simulink model "boost_ms"  (R2020b)
settings: Solver=VariableStepAuto  StartTime=0.0  StopTime=10.0  RelTol=1e-3
libraries: powerlib x10, powerlib_meascontrol x3, re_lib x1
settings Model: Creator=mcapuano  LastModifiedBy=mcapuano

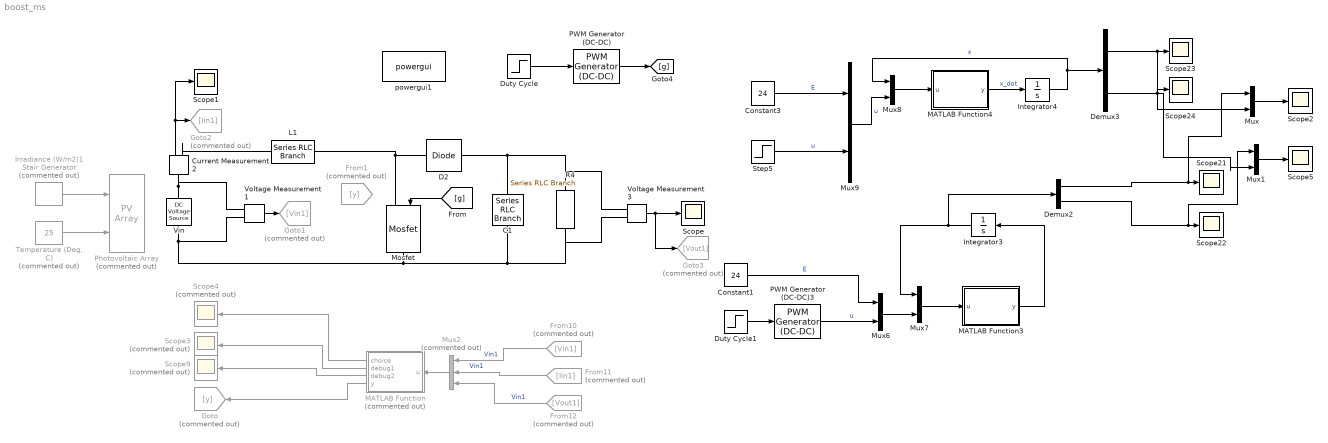
== system boost_ms ==
  C1 : powerlib/Elements/Series RLC Branch  LConnTagsString=__new0  RConnTagsString=__new0  BranchType=C  Resistance=1e-4  Inductance=200e-6  SetiL0=off  InitialCurrent=0  Capacitance=200e-6  Setx0=on  InitialVoltage=0  Measurements=None
  Constant1 : Constant  Value=24
  Constant3 : Constant  Value=24
  Current Measurement2 : powerlib/Measurements/Current Measurement  PhasorSimulation=off  OutputType=Complex  PSBequivalent=0
  D2 : powerlib/Power Electronics/Diode  Ron=1e-3  Lon=0  Vf=0  IC=0  UseSnubber=off  Rs=inf  Cs=inf  Measurements=off
  Demux2 : Demux  Outputs=2
  Demux3 : Demux  Outputs=2
  Duty Cycle : Step  Time=.5  Before=.5  After=.5  SampleTime=0
  Duty Cycle1 : Step  Time=.1  Before=.5  After=.5  SampleTime=0
  From1 : From  Commented=on  GotoTag=y
  From10 : From  Commented=on  GotoTag=Vin1
  From11 : From  Commented=on  GotoTag=Iin1
  From12 : From  Commented=on  GotoTag=Vout1
  Goto : Goto  Commented=on  GotoTag=y
  Goto1 : Goto  Commented=on  GotoTag=Vin1
  Goto2 : Goto  Commented=on  GotoTag=Iin1
  Goto3 : Goto  Commented=on  GotoTag=Vout1
  Integrator3 : Integrator  InitialCondition=[0 0]
  Integrator4 : Integrator  InitialCondition=[0 0]
  Irradiance (W/m2)1 : powerlib_meascontrol/Pulse & Signal Generators/Stair Generator  Commented=on  t=[0, 0.5, 1, 1.5, 2]  e=[0.5, 0.7, 0.8, 0.6, 0.2]*1000  Ts=15e-6
  L1 : powerlib/Elements/Series RLC Branch  LConnTagsString=__new0  RConnTagsString=__new0  BranchType=L  Resistance=1e-4  Inductance=250e-6  SetiL0=on  InitialCurrent=0  Capacitance=30e-6  Setx0=off  InitialVoltage=150  Measurements=None
  MATLAB Function : MATLAB Function  Commented=on  TreatAsAtomicUnit=on  SystemSampleTime=15e-6
  MATLAB Function3 : MATLAB Function  TreatAsAtomicUnit=on
  MATLAB Function4 : MATLAB Function  TreatAsAtomicUnit=on
  Mosfet : powerlib/Power Electronics/Mosfet  Ron=1e-3  Lon=0  Rd=1e-3  Vfd=0  IC=0  Rs=1e6  Cs=inf  Measurements=off
  Mux{,1,6..9} (6 alike) : Mux  Inputs=2
  Mux2 : Mux  Commented=on  Inputs=3
  PWM Generator (DC-DC) : powerlib_meascontrol/Pulse & Signal Generators/PWM Generator (DC-DC)  Fsw=66.67e3  Ts=0
  PWM Generator (DC-DC)3 : powerlib_meascontrol/Pulse & Signal Generators/PWM Generator (DC-DC)  Fsw=66.67e3  Ts=0
  Photovoltaic Array : re_lib/Solar/PV Array  Commented=on  Npar=1  Nser=1  PlotType=one module @ 25 deg.C & specified irradiances  S_vec=[800]  Temp_C_vec=[ 50 ]  ModuleName=Kyocera Solar KC200GT  PlotWhenSelected=off  Pm=200.143  Ncell=54  Voc=32.9  Isc=8.21  Vm=26.3  Im=7.61  beta_Voc_pc=-0.355  alpha_Isc_pc=0.06  beta_Voc=-0.11679  alpha_Isc=0.004926  IL=8.2288  I0=2.3234e-10  nI=0.97734  Rsh=150.6844  Rs=0.34484  RobustModel=off  RobustCellTemperature=313.3991  BAL=on  Tc=1e-6  Tfilter=5e-5
      settings: AttributesFormatString=|
      | %<ModuleName>
      | %<Nser>-module string
      | %<Npar> parallel strings
  R4 : powerlib/Elements/Series RLC Branch  LConnTagsString=__new0  RConnTagsString=__new0  BranchType=R  Resistance=3  Inductance=200e-6  SetiL0=off  InitialCurrent=0  Capacitance=400e-6  Setx0=off  InitialVoltage=0  Measurements=None
  Scope{,1..2,5,21..24} (8 alike) : Scope
  Scope3 : Scope  Commented=on
  Scope4 : Scope  Commented=on
  Scope9 : Scope  Commented=on
  Step5 : Step  Time=.1  Before=.5  After=.5  SampleTime=0
  Temperature (Deg. C) : Constant  Commented=on  Value=25
  Vin : powerlib/Electrical Sources/DC Voltage Source  Amplitude=24  Measurements=None
  Voltage Measurement1 : powerlib/Measurements/Voltage Measurement  PhasorSimulation=off  OutputType=Complex  PSBequivalent=0
  Voltage Measurement3 : powerlib/Measurements/Voltage Measurement  PhasorSimulation=off  OutputType=Complex  PSBequivalent=0
  powergui1 : powerlib/powergui  Priority=1  SimulationMode=Continuous  SampleTime=50e-6  frequency=60  Iterations=50  frequencyindice=0  Pbase=100e6  ErrMax=1e-4  UnitsV=kV  UnitsW=MW  buscounter=0  FunctionMessages=off  echomessages=off  EnableUseOfTLC=off  CurrentSourceSwitches=off  DisableSnubberDevices=off  DisableRonSwitches=off  DisableVfSwitches=off  DisplayEquations=off  AutomaticDiscreteSolvers=off  SolverType=Tustin/Backward Euler (TBE)  Interpol=off  ExternalGateDelay=off  methode=off  Ts=100  x0status=blocks  SPID=on  SwTol=0  HookPort=off  NonlinearTolerance=1e-4  nMaxIteration=100  ContinueOnMaxIteration=off  RestoreLinks=warning  ResistiveCurrentMeasurement=off  Frange=[0:2:500]  Ylog=off  Xlog=on  ShowGrid=off  save=off  variable=ZData  structure=0  ZoomFFT=off  StartTime=0.0  cycles=1  DisplayStyle=1  fundamental=60  FreqAxis=off  MaxFrequency=1000  frequencyindicesteady=1  RmsSteady=1  display=off
  wires:
  PWM Generator (DC-DC)/1 -> [g]
  Duty Cycle/1 -> PWM Generator (DC-DC)/1
  [g] -> Mosfet/1
  Voltage Measurement3/1 -> Goto3/1, Scope/1
  Temperature (Deg. C)/1 -> Photovoltaic Array/2
  Irradiance (W/m2)1/1 -> Photovoltaic Array/1
  MATLAB Function/3(debug2) -> Scope9/1
  From11/1 -> Mux2/2  "Vin1"
  MATLAB Function/2(debug1) -> Scope3/1
  MATLAB Function/1(choice) -> Scope4/1
  From10/1 -> Mux2/1  "Vin1"
  Mux2/1 -> MATLAB Function/1(u)
  From12/1 -> Mux2/3  "Vin1"
  MATLAB Function/4(y) -> Goto/1
  Voltage Measurement1/1 -> Goto1/1
  Current Measurement2/1 -> Scope1/1, Goto2/1
  Mux9/1 -> Mux8/2  "u"
  Constant3/1 -> Mux9/1  "E"
  Demux2/2 -> Mux1/1, Scope22/1
  PWM Generator (DC-DC)3/1 -> Mux6/2  "u"
  Mux8/1 -> MATLAB Function4/1(u)
  Integrator3/1 -> Demux2/1, Mux7/1
  Demux3/1 -> Mux/2, Scope23/1
  Mux7/1 -> MATLAB Function3/1(u)
  Integrator4/1 -> Mux8/1, Demux3/1  "x"
  Demux3/2 -> Mux1/2, Scope24/1
  Mux6/1 -> Mux7/2
  Demux2/1 -> Mux/1, Scope21/1
  Duty Cycle1/1 -> PWM Generator (DC-DC)3/1
  MATLAB Function4/1(y) -> Integrator4/1  "x_dot"
  MATLAB Function3/1(y) -> Integrator3/1
  Constant1/1 -> Mux6/1  "E"
  Step5/1 -> Mux9/2  "u"
  Mux/1 -> Scope2/1
  Mux1/1 -> Scope5/1
  connections:
  Vin/RConn1 -- Voltage Measurement1/LConn1 -- Current Measurement2/LConn1
  Vin/LConn1 -- Voltage Measurement1/LConn2 -- Voltage Measurement3/LConn2 -- R4/RConn1 -- C1/RConn1 -- Mosfet/RConn1
  L1/RConn1 -- Mosfet/LConn1 -- D2/LConn1
  D2/RConn1 -- Voltage Measurement3/LConn1 -- R4/LConn1 -- C1/LConn1
  Current Measurement2/RConn1 -- L1/LConn1

== matlab function boost_ms/MATLAB Function ==
  settings: updateMethod=DISCRETE
  data: choice output; debug1 output; debug2 output; u input; y output
function [choice, debug1, debug2, y]= fcn(u)
Vpv=u(1);
Ipv=u(2);
Vout=u(3);

%This module contains the MPC-MPPT Control Algorithm

%The MPC module follows the flow chart of Fig. 8 in Referenced Research Paper

%This MATLAB fn block's settings have been changed to have a sampling rate
%of 15uS instead of being continous sample mode


%prevent crazy simulation transients from breaking the algorithm:
if (Ipv > 10)
    Ipv = 1;
end

persistent Vpv_t_1; %previous Vpv Sample
if isempty(Vpv_t_1)
    Vpv_t_1 = 0;
end
persistent Ipv_t_1; %previous Ipv Sample
if isempty(Ipv_t_1)
    Ipv_t_1 = 0;
end
persistent Dpv_t_1; % Iref (output) value from what is now 2 timesteps ago
if isempty(Dpv_t_1)
    Dpv_t_1 = 0;
end
persistent Dpv;  %Previous / Most recent Iref (output) Calc
if isempty(Dpv)
    Dpv = 0;
end

Ts = 15e-6; %sample rate
L = 3e-3; %inductance


delta_V = Vpv - Vpv_t_1;
delta_I = Ipv - Ipv_t_1;
delta_D = Dpv - Dpv_t_1;


%fixed vs adaptive
scale_factor_C = 10; %increase for larger output increments/swings
 Z =.01; %fixed 
%Z = scale_factor_C * abs(delta_I * delta_D); %adaptive

% custom adaptive to fix issues with no change causing 0 step size
 adapZ = scale_factor_C * abs(delta_I * delta_D);
% if(adapZ > .1)
%     Z = .1;
% elseif(adapZ > .001)
%     Z = adapZ;
% else
%     Z = .001;
% end

Ipred_1 = Ipv + 2*(Ts/L) * Vpv; %MPC prediction for switch = 1
Ipred_0 = Ipv + (Ts/(2*L)* (Vpv - Vout)); %MPC prediction for switch = 0 

if delta_V == 0 %Inc. Cond. Algo to determin Iref
    if delta_I == 0 
        Iref = Dpv; choice = 0;
    else
        if delta_I > 0
            Iref = Dpv - Z; choice = 1;
        else
            Iref = Dpv + Z; choice = 2;
        end
    end
else
    if (Ipv + (delta_I/delta_V) * Vpv) == 0
        Iref = Dpv; choice = 3;
    else
        if (Ipv + (delta_I/delta_V) * Vpv) > 0
            Iref = Dpv - Z; choice = 4;
        else
            Iref = Dpv + Z; choice = 5;
        end
    end
end

G1 = abs(Iref - Ipred_1); %Optimize MPC by applying Iref
G0 = abs(Iref - Ipred_0);
if G1 < G0
    y = 1;
else
    y = 0;
end

if (Iref < 0)
    Iref = .001;
end
%test = Ipv + (delta_I/delta_V) * Vpv;
test =  delta_V;
%update static variables here:
Vpv_t_1 = Vpv; %previous Vpv Sample
Ipv_t_1 = Ipv; %previous Ipv Sample
Dpv_t_1 = Dpv; % Iref (output) value from what is now 2 timesteps ago
Dpv = Iref;  %Previous / Most recent Iref (output) Calc

%debug purposes:
debug1 = Vout;
debug2 = delta_I/delta_V;

== matlab function boost_ms/MATLAB Function3 ==
  data: u input; y output
function y = fcn(u)
X=u(1:2);
E=u(3);
u=u(4);
% parameters:
C=200e-6;
L=250e-6;
R=3;

% Compact form
A=[ 0    -1/L ;
   1/C  -1/(C*R)];

B=[0   1/L;
   -1/C  0];

b=[0; 0];

d=[E/L; 0];

y = A*X+(B*X+ b)*u+d;

== matlab function boost_ms/MATLAB Function4 ==
  data: u input; y output
function y = fcn(u)

X=u(1:2);
E=u(3);
u=u(4);
% parameters:
C=200e-6;
L=250e-6;
R=3;

%%%begin PWM detector
% persistent D; 
% if isempty(D)
%     D = 0;
% end
% 
% persistent T_on; 
% if isempty(T_on)
%     T_on = 0;
% end
% 
% persistent T_off; 
% if isempty(T_off)
%     T_off = 0;
% end
% 
% persistent u_prev; 
% if isempty(u_prev)
%     u_prev = 0;
% end
% 
% persistent Ts; 
% if isempty(Ts)
%     Ts = 0;
% end
% 
% if(u_prev == 0 && u == 1)
%     D = T_on / Ts;
%     Ts = 15e-6;
%     T_on = 15e-6;
%     T_off = 0;
% else
%     D = D;
%     if(u == 1)
%     Ts = Ts + 15e-6;
%     T_on = T_on + 15e-6;
%     else
%      Ts = Ts + 15e-6;
%      T_off = T_off + 15e-6;
%     end
% end
% 
% 
% 
% u_prev = u;
%%%end PWM detector
D = .5;

A=[ 0    (-1+D)/L ;
   (1-D)/C  -1/(C*R)];

B=[1/L;
   0];

u = E;

 y = A*X+B*u;
